simulink model "exemplar"  (R2023b)
settings: Solver=ode45  StartTime=0.0  StopTime=240  MaxStep=1  RelTol=1e-3
libraries: F3M_commonLib x7
PreSaveFcn:
  | MakeLibLight();
settings Model: Creator=nshoman  LastModifiedBy=nshoman
settings DataIOCC: SaveOutput=off  SignalLogging=off  DSMLogging=off  SaveTime=off  ReturnWorkspaceOutputs=off

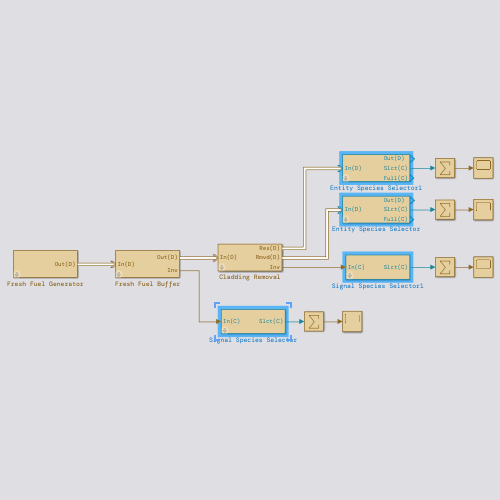
[thumbnail: Simulink's stored preview of the top-level diagram]
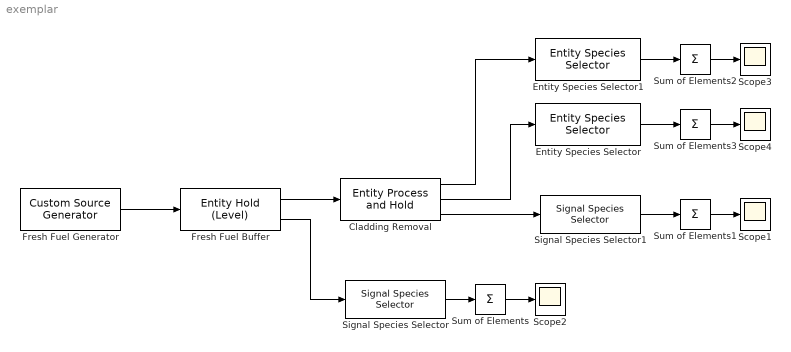
== system exemplar ==
  Cladding Removal : F3M_commonLib/Entity Process and Hold  t_process=5  ptable={ 'all', '0.99'; 'U', '0'; 'O', '0' }
      settings: SourceProductName=Fissile Facility Flow Modeler
  Entity Species Selector : F3M_commonLib/Entity Species Selector  InString=fe  width=0.10
      settings: SourceProductName=Fissile Facility Flow Modeler
  Entity Species Selector1 : F3M_commonLib/Entity Species Selector  InString=fe  width=0.10
      settings: SourceProductName=Fissile Facility Flow Modeler
  Fresh Fuel Buffer : F3M_commonLib/Entity Hold (Level)  nitems=2  time=30
      settings: SourceProductName=Fissile Facility Flow Modeler
  Fresh Fuel Generator : F3M_commonLib/Custom Source Generator  size=250  period=30  ptable={ 'U', '0.40'; 'O', '0.20'; 'C', '0.00012'; 'Cr', '0.072'; 'Mn', '0.008'; 'Ni', '0.032'; 'N', '0.004'; 'P', '0.00018'; 'Si', '0.003'; 'S', '0.00012'; 'Fe', '0.28148' }
      settings: SourceProductName=Fissile Facility Flow Modeler
  Scope{1..4} (4 alike) : Scope
  Signal Species Selector : F3M_commonLib/Signal Species Selector  InString=u
      settings: SourceProductName=Fissile Facility Flow Modeler
  Signal Species Selector1 : F3M_commonLib/Signal Species Selector  InString=u
      settings: SourceProductName=Fissile Facility Flow Modeler
  Sum of Elements{,1..3} (4 alike) : Sum  Inputs=+
  wires:
  Fresh Fuel Generator/1 -> Fresh Fuel Buffer/1
  Fresh Fuel Buffer/1 -> Cladding Removal/1
  Fresh Fuel Buffer/2 -> Signal Species Selector/1
  Signal Species Selector/1 -> Sum of Elements/1
  Sum of Elements/1 -> Scope2/1
  Sum of Elements1/1 -> Scope1/1
  Signal Species Selector1/1 -> Sum of Elements1/1
  Cladding Removal/3 -> Signal Species Selector1/1
  Sum of Elements2/1 -> Scope3/1
  Cladding Removal/1 -> Entity Species Selector1/1
  Entity Species Selector1/2 -> Sum of Elements2/1
  Entity Species Selector/2 -> Sum of Elements3/1
  Sum of Elements3/1 -> Scope4/1
  Cladding Removal/2 -> Entity Species Selector/1
